simulink model "parcial_20241125"  (R2021a)
settings: Solver=ode4  StartTime=0.0  StopTime=10.0  FixedStep=0.0001  RelTol=1e-3
libraries: cstblocks x2
settings Model: Creator=aghersin  LastModifiedBy=frand
settings SolverCC: AlgebraicLoopSolver=TrustRegion
settings DataIOCC: ReturnWorkspaceOutputs=off
settings OptimizationCC: LifeSpan=inf
settings DebuggingCC: SFExecutionAtInitializationDiag=none  SFMachineParentedDataDiag=warning  ArithmeticOperatorsInVariantConditions=warning
settings SFSimCC: SimUseLocalCustomCode=off  CustomCodeUndefinedFunction=UseInterfaceOnly
settings RTWCC: RTWUseLocalCustomCode=off
settings CodeAppCC: StateflowObjectComments=on

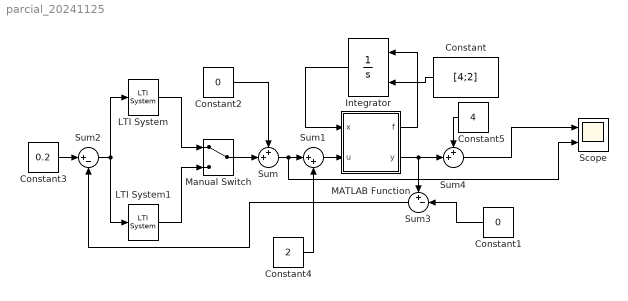
== system parcial_20241125 ==
  Constant : Constant  Value=[4;2]
  Constant1 : Constant  Value=0
  Constant2 : Constant  Value=0
  Constant3 : Constant  Value=0.2
  Constant4 : Constant  Value=2
  Constant5 : Constant  Value=4
  Integrator : Integrator  InitialConditionSource=external
  LTI System : cstblocks/LTI System  sys=C_digit  IC=[]
  LTI System1 : cstblocks/LTI System  sys=C  IC=[]
  MATLAB Function : MATLAB Function  TreatAsAtomicUnit=on
  Manual Switch : ManualSwitch
  Scope : Scope  NumInputPorts=2
  Sum : Sum  Inputs=++|
  Sum1 : Sum  Inputs=|++
  Sum2 : Sum  Inputs=|+-
  Sum3 : Sum  Inputs=+-|
  Sum4 : Sum  Inputs=++|
  wires:
  Integrator/1 -> MATLAB Function/1(x)
  MATLAB Function/1(f) -> Integrator/1
  Constant/1 -> Integrator/2
  MATLAB Function/2(y) -> Sum4/2, Sum3/1
  Constant1/1 -> Sum3/2
  Constant2/1 -> Sum/1
  Sum2/1 -> LTI System1/1, LTI System/1
  Constant3/1 -> Sum2/1
  Sum3/1 -> Sum2/2
  Sum/1 -> Scope/2, Sum1/1
  Sum1/1 -> MATLAB Function/2(u)
  Constant4/1 -> Sum1/2
  Sum4/1 -> Scope/1
  Constant5/1 -> Sum4/1
  LTI System1/1 -> Manual Switch/2
  LTI System/1 -> Manual Switch/1
  Manual Switch/1 -> Sum/2

== matlab function parcial_20241125/MATLAB Function ==
  data: x input; u input; f output; y output
function [f,y] = fcn(x,u)

f1=(x(2)-sqrt(x(1)))/x(1)^2;
f2=4*u-4*x(2);

f=[f1;f2];

y=x(1)^(-3/2);
